simulink model "CEL_Lab1_Simulink"  (R2023b)
settings: Solver=VariableStepAuto  StartTime=0.0  StopTime=5
values from neighbouring files (symbols this model uses):
  k_d = 0    [Start_upSimulinkModel.m]    (also in load_params_inertial_case.m)
  k_i = 2    [Start_upSimulinkModel.m]    (also in load_params_inertial_case.m = 0)
  k_p = 10    [Start_upSimulinkModel.m]    (also in load_params_inertial_case.m = 3)
  rads2rpm = 60/2/pi    (= 9.54929658551)    [load_params_inertial_case.m]
  T_l = 0.001    [Start_upSimulinkModel.m]    (also in load_params_inertial_case.m)
undefined symbols (not defined in the file or in its folder): drv, gbox, mld, mot, sens
libraries: simulink_extras x3
settings Model: Creator=bmm1  LastModifiedBy=bmm1
settings SolverCC: ZeroCrossControl=DisableAll

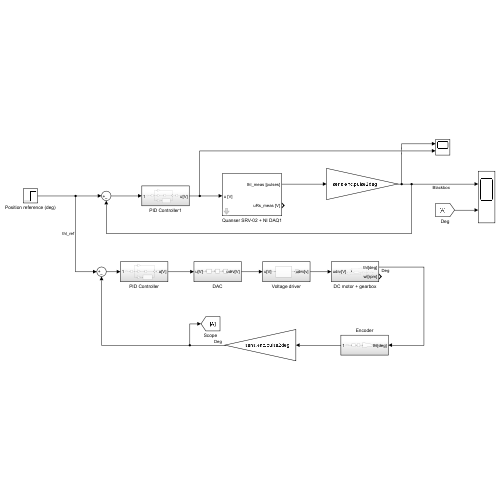
[thumbnail: Simulink's stored preview of the top-level diagram]
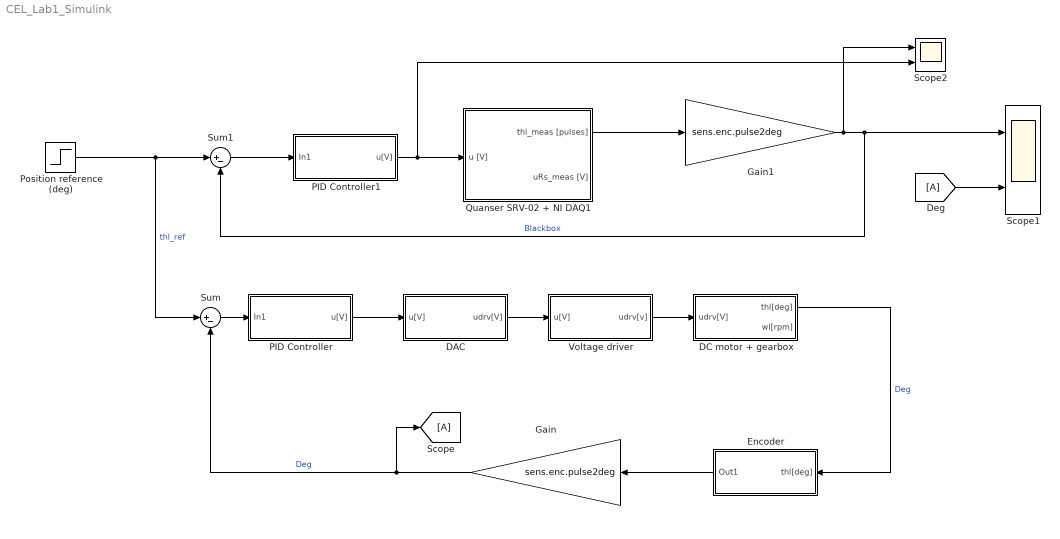
== system CEL_Lab1_Simulink ==
  DAC : Subsystem
  DC motor + gearbox : Subsystem
  Deg : From
  Encoder : Subsystem
  Gain : Gain  Gain=sens.enc.pulse2deg
  Gain1 : Gain  Gain=sens.enc.pulse2deg
  PID Controller : Subsystem
  PID Controller1 : Subsystem
  Position reference (deg) : Step  Time=0.5  After=20  SampleTime=0
  Quanser SRV-02 + NI DAQ1 : Subsystem  mask(Quanser SRV-02 (with inertial load) + NI DAQ){Ts=0.001, fricType=Coulomb + viscous}
      mask prompts: Ts "NI DAQ Sample Time:"; fricType "Friction model"
      mask help: Quanser SRV-02 (with inertial load) + NI DAQ model.
      mask init:
      | %%  Sensors data
      | 
      | %   shunt resistor
      | sens.curr.Rs = 0.5;                         %   resistance [Ohm]   
      | sens.curr.uRs_std = 0.01;                   %   voltage noise standard dev [V]                           
      | sens.curr.uRs_var = sens.curr.uRs_std^2;	%   voltage noise variance [V^2]
      | 
      | %   Hewlett-Packard HEDS-5540#A06 optical encoder
      | sens.enc.ppr = 500*4;                       %   pulses per rotation
      | sens.enc.pulse2deg = 360/sens.enc.ppr;      %   [pulses] -> [deg]
      | sens.enc.pulse2rad = 2*pi/sens.enc.ppr;     %   [pulses] -> [rad]
      | sens.enc.deg2pulse = sens.enc.ppr/360;      %   [deg] -> [pulses]
      | sens.enc.rad2pulse = sens.enc.ppr/2/pi;     %   [rad] -> [pulses]
      | 
      | 
      | %%  Data acquisition board (daq) data
      | 
      | %   NI PCI-6221 DAC data
      | daq.dac.bits = 16;                                  %   resolution (bits)
      | daq.dac.fs   = 10;                                  %   full scale 
      | daq.dac.q    = 2*daq.dac.fs/(2^daq.dac.bits-1);     %	quantization
      | 
      | %   NI PCI-6221 ADC data
      | daq.adc.bits = 16;                                  %   resolution (bits)
      | daq.adc.fs   = 10;                                  %   full scale (as set in SLDRT Analog Input block)
      | daq.adc.q    = 2*daq.adc.fs/(2^daq.adc.bits-1);     %   quantization
      mask Help:
      | Riccardo Antonello (antonello@dei.unipd.it)
      | 
      | April 24, 2020
      | 
      | Dept. of Information Engineering, University of Padova
      mask TypeOptions fricType: Coulomb + viscous | Karnopp
  Scope : Goto
  Scope1 : Scope  NumInputPorts=2
  Scope2 : Scope  NumInputPorts=2
  Sum : Sum  Inputs=|+-
  Sum1 : Sum  Inputs=|+-
  Voltage driver : Subsystem
  wires:
  Position reference (deg)/1 -> Sum/1, Sum1/1  "thl_ref"
  Gain/1 -> Sum/2, Scope/1  "Deg"
  Sum/1 -> PID Controller/1(In1)
  PID Controller/1(u[V]) -> DAC/1(u[V])
  DAC/1(udrv[V]) -> Voltage driver/1(u[V])
  Voltage driver/1(udrv[v]) -> DC motor + gearbox/1(udrv[V])
  DC motor + gearbox/1(thl[deg]) -> Encoder/1(thl[deg])  "Deg"
  Quanser SRV-02 + NI DAQ1/1(thl_meas [pulses]) -> Gain1/1
  Gain1/1 -> Scope2/1, Sum1/2, Scope1/1  "Blackbox"
  PID Controller1/1(u[V]) -> Scope2/2, Quanser SRV-02 + NI DAQ1/1(u [V])
  Sum1/1 -> PID Controller1/1(In1)
  Encoder/1(Out1) -> Gain/1
  Deg/1 -> Scope1/2

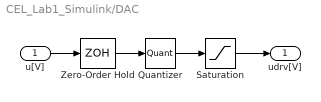
== system CEL_Lab1_Simulink/DAC ==
  u[V] : Inport
  Quantizer : Quantizer  QuantizationInterval=daq.dac.q
  Saturation : Saturate  UpperLimit=10  LowerLimit=-10
  Zero-Order Hold : ZeroOrderHold  SampleTime=1e-3
  udrv[V] : Outport
  wires:
  Zero-Order Hold/1 -> Quantizer/1
  u[V]/1 -> Zero-Order Hold/1
  Quantizer/1 -> Saturation/1
  Saturation/1 -> udrv[V]/1

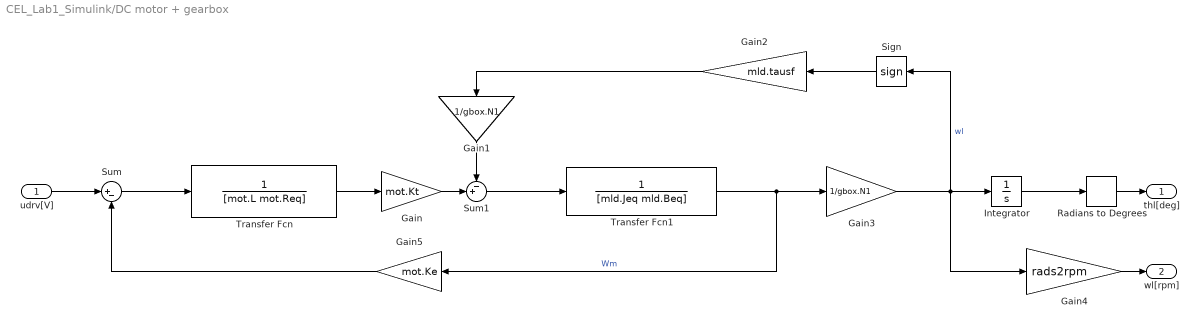
== system CEL_Lab1_Simulink/DC motor + gearbox ==
  udrv[V] : Inport
  Gain : Gain  Gain=mot.Kt
  Gain1 : Gain  Gain=1/gbox.N1
  Gain2 : Gain  Gain=mld.tausf
  Gain3 : Gain  Gain=1/gbox.N1
  Gain4 : Gain  Gain=rads2rpm
  Gain5 : Gain  Gain=mot.Ke
  Integrator : Integrator
  Radians to Degrees : simulink_extras/Transformations/Radians to Degrees
  Sign : Signum
  Sum : Sum  Inputs=|+-
  Sum1 : Sum  Inputs=-+|
  Transfer Fcn : TransferFcn  Denominator=[mot.L mot.Req]
  Transfer Fcn1 : TransferFcn  Denominator=[mld.Jeq mld.Beq]
  thl[deg] : Outport
  wl[rpm] : Outport  Port=2
  wires:
  udrv[V]/1 -> Sum/1
  Sum/1 -> Transfer Fcn/1
  Transfer Fcn/1 -> Gain/1
  Gain1/1 -> Sum1/1
  Gain2/1 -> Gain1/1
  Sign/1 -> Gain2/1
  Transfer Fcn1/1 -> Gain5/1, Gain3/1  "Wm"
  Gain3/1 -> Gain4/1, Sign/1, Integrator/1  "wl"
  Integrator/1 -> Radians to Degrees/1
  Radians to Degrees/1 -> thl[deg]/1
  Gain4/1 -> wl[rpm]/1
  Sum1/1 -> Transfer Fcn1/1
  Gain/1 -> Sum1/2
  Gain5/1 -> Sum/2

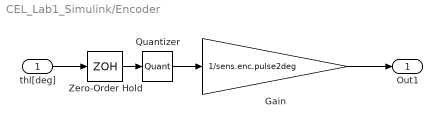
== system CEL_Lab1_Simulink/Encoder ==
  thl[deg] : Inport
  Gain : Gain  Gain=1/sens.enc.pulse2deg
  Quantizer : Quantizer  QuantizationInterval=sens.enc.pulse2deg
  Zero-Order Hold : ZeroOrderHold  SampleTime=1e-3
  Out1 : Outport
  wires:
  thl[deg]/1 -> Zero-Order Hold/1
  Gain/1 -> Out1/1
  Quantizer/1 -> Gain/1
  Zero-Order Hold/1 -> Quantizer/1

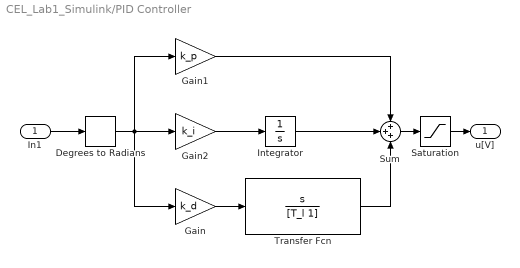
== system CEL_Lab1_Simulink/PID Controller ==
  In1 : Inport
  Degrees to Radians : simulink_extras/Transformations/Degrees to Radians
  Gain : Gain  Gain=k_d
  Gain1 : Gain  Gain=k_p
  Gain2 : Gain  Gain=k_i
  Integrator : Integrator
  Saturation : Saturate  UpperLimit=10  LowerLimit=-10
  Sum : Sum  Inputs=+++
  Transfer Fcn : TransferFcn  Numerator=[1 0]  Denominator=[T_l 1]
  u[V] : Outport
  wires:
  In1/1 -> Degrees to Radians/1
  Sum/1 -> Saturation/1
  Saturation/1 -> u[V]/1
  Degrees to Radians/1 -> Gain/1, Gain1/1, Gain2/1
  Gain/1 -> Transfer Fcn/1
  Gain2/1 -> Integrator/1
  Transfer Fcn/1 -> Sum/3
  Integrator/1 -> Sum/2
  Gain1/1 -> Sum/1

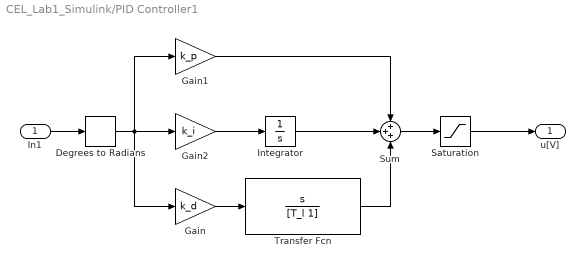
== system CEL_Lab1_Simulink/PID Controller1 ==
  In1 : Inport
  Degrees to Radians : simulink_extras/Transformations/Degrees to Radians
  Gain : Gain  Gain=k_d
  Gain1 : Gain  Gain=k_p
  Gain2 : Gain  Gain=k_i
  Integrator : Integrator
  Saturation : Saturate  UpperLimit=10  LowerLimit=-10
  Sum : Sum  Inputs=+++
  Transfer Fcn : TransferFcn  Numerator=[1 0]  Denominator=[T_l 1]
  u[V] : Outport
  wires:
  In1/1 -> Degrees to Radians/1
  Sum/1 -> Saturation/1
  Saturation/1 -> u[V]/1
  Degrees to Radians/1 -> Gain/1, Gain1/1, Gain2/1
  Gain/1 -> Transfer Fcn/1
  Gain2/1 -> Integrator/1
  Transfer Fcn/1 -> Sum/3
  Integrator/1 -> Sum/2
  Gain1/1 -> Sum/1

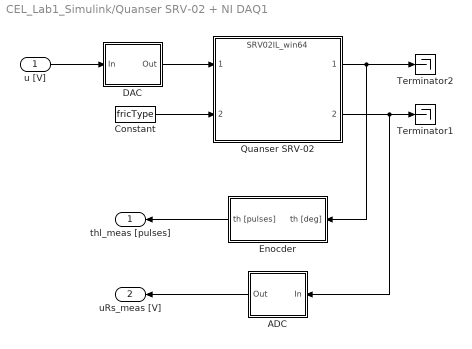
== system CEL_Lab1_Simulink/Quanser SRV-02 + NI DAQ1 ==
  u [V] : Inport
  ADC : Subsystem
  Constant : Constant  Value=fricType
  DAC : Subsystem
  Enocder : Subsystem
  Quanser SRV-02 : ModelReference  ModelNameDialog=SRV02IL_win64.slxp  ModelReferenceVersion=1.44  CopyOfModelProtected=on
  Terminator1 : Terminator
  Terminator2 : Terminator
  thl_meas [pulses] : Outport
  uRs_meas [V] : Outport  Port=2
  wires:
  Enocder/1(th [pulses]) -> thl_meas [pulses]/1
  ADC/1(Out) -> uRs_meas [V]/1
  DAC/1(Out) -> Quanser SRV-02/1
  Quanser SRV-02/2 -> ADC/1(In), Terminator1/1
  u [V]/1 -> DAC/1(In)
  Quanser SRV-02/1 -> Enocder/1(th [deg]), Terminator2/1
  Constant/1 -> Quanser SRV-02/2

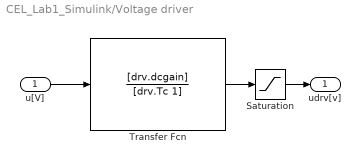
== system CEL_Lab1_Simulink/Voltage driver ==
  u[V] : Inport
  Saturation : Saturate  UpperLimit=12  LowerLimit=-12
  Transfer Fcn : TransferFcn  Numerator=[drv.dcgain]  Denominator=[drv.Tc 1]
  udrv[v] : Outport
  wires:
  u[V]/1 -> Transfer Fcn/1
  Transfer Fcn/1 -> Saturation/1
  Saturation/1 -> udrv[v]/1

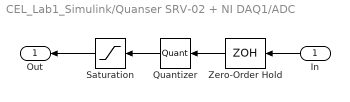
== system CEL_Lab1_Simulink/Quanser SRV-02 + NI DAQ1/ADC ==
  In : Inport
  Quantizer : Quantizer  QuantizationInterval=daq.adc.q
  Saturation : Saturate  UpperLimit=daq.adc.fs  LowerLimit=-daq.adc.fs
  Zero-Order Hold : ZeroOrderHold  SampleTime=Ts
  Out : Outport
  wires:
  Saturation/1 -> Out/1
  In/1 -> Zero-Order Hold/1
  Quantizer/1 -> Saturation/1
  Zero-Order Hold/1 -> Quantizer/1

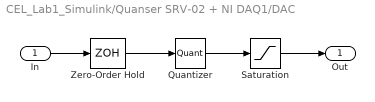
== system CEL_Lab1_Simulink/Quanser SRV-02 + NI DAQ1/DAC ==
  In : Inport
  Quantizer : Quantizer  QuantizationInterval=daq.dac.q
  Saturation : Saturate  UpperLimit=daq.dac.fs  LowerLimit=-daq.dac.fs
  Zero-Order Hold : ZeroOrderHold  SampleTime=Ts
  Out : Outport
  wires:
  Quantizer/1 -> Saturation/1
  In/1 -> Zero-Order Hold/1
  Zero-Order Hold/1 -> Quantizer/1
  Saturation/1 -> Out/1

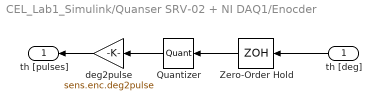
== system CEL_Lab1_Simulink/Quanser SRV-02 + NI DAQ1/Enocder ==
  th [deg] : Inport
  Quantizer : Quantizer  QuantizationInterval=sens.enc.pulse2deg
  Zero-Order Hold : ZeroOrderHold  SampleTime=Ts
  deg2pulse : Gain  Gain=sens.enc.deg2pulse
  th [pulses] : Outport
  wires:
  Quantizer/1 -> deg2pulse/1
  th [deg]/1 -> Zero-Order Hold/1
  Zero-Order Hold/1 -> Quantizer/1
  deg2pulse/1 -> th [pulses]/1
